simulink model "FlightModel"  (R2024b)
settings: Solver=ode1  StartTime=0.0  StopTime=inf  FixedStep=sampletime  RelTol=1e-3
values from neighbouring files (symbols this model uses):
  g = 9.807    [start.m]
undefined symbols (not defined in the file or in its folder): INI
settings Model: Creator=Nguewo  LastModifiedBy=annaf
settings SolverCC: AlgebraicLoopSolver=TrustRegion
settings DebuggingCC: UnconnectedInputMsg=warning  UnconnectedOutputMsg=warning  UnconnectedLineMsg=warning
settings ModelReferenceCC: EnableRefExpFcnMdlSchedulingChecks=on
settings RTWCC: GPUComputeCapability=3.5  DLArmComputeVersion=19.05

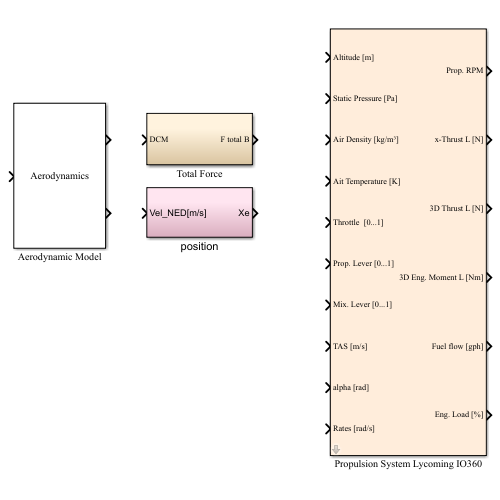
[thumbnail: Simulink's stored preview of the top-level diagram]
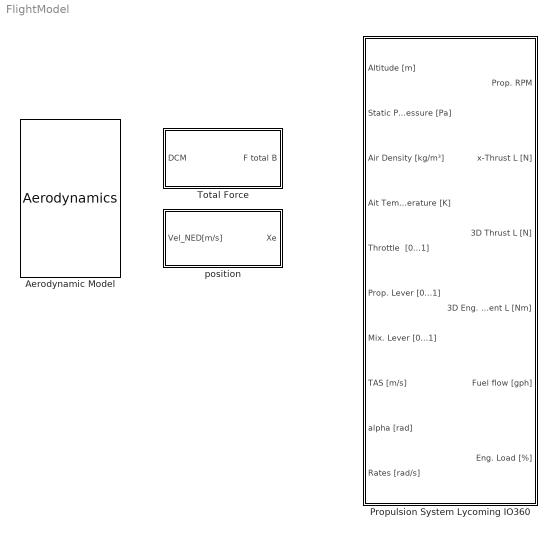
== system FlightModel ==
  Aerodynamic Model : M-S-Function  FunctionName=Aerodynamics
  Propulsion System Lycoming IO360 : Subsystem  mask{Y_TW=0}
      mask prompts: Y_TW "Y Position of the Engine [m]. Positive for Left Engine"
  Total Force : Subsystem
  position : Subsystem

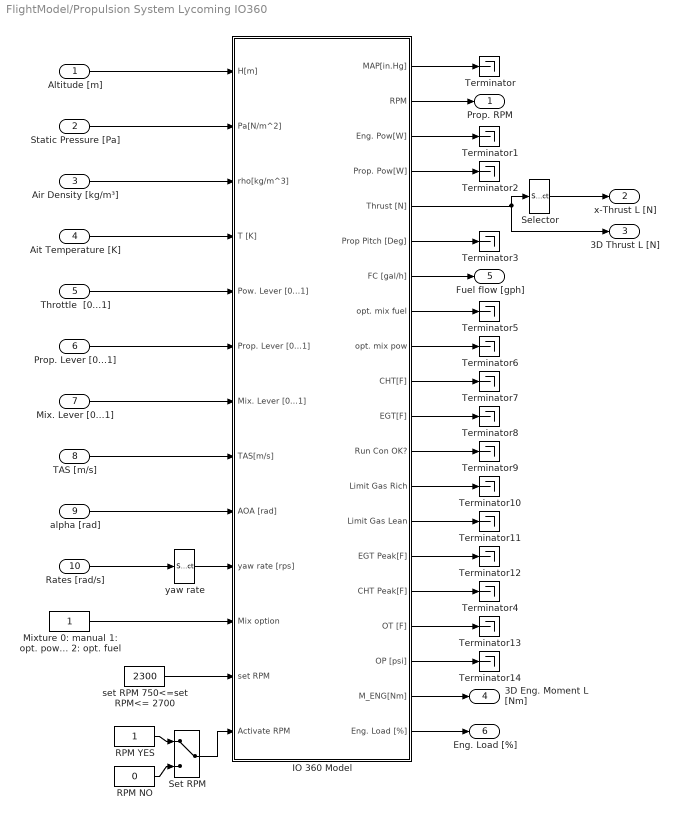
== system FlightModel/Propulsion System Lycoming IO360 ==
  Altitude [m] : Inport
  Static Pressure [Pa] : Inport  Port=2
  Air Density [kg/m³] : Inport  Port=3
  Ait Temperature [K] : Inport  Port=4
  Throttle  [0...1] : Inport  Port=5
  Prop. Lever [0...1] : Inport  Port=6
  Mix. Lever [0...1] : Inport  Port=7
  TAS [m/s] : Inport  Port=8
  alpha [rad] : Inport  Port=9
  Rates [rad/s] : Inport  Port=10
  IO 360 Model : Subsystem
  "Mixture 0: manual 1: opt. pow 2: opt. fuel " : Constant
  RPM NO : Constant  Value=0
  RPM YES : Constant
  Selector : Selector  InputPortWidth=3  IndexOptions=Index vector (dialog)  Indices=1  OutputSizes=1
  Set RPM : ManualSwitch
  Terminator{,1..14} (15 alike) : Terminator
  set RPM 750<=set RPM<= 2700 : Constant  Value=2300
  yaw rate : Selector  InputPortWidth=3  IndexOptions=Index vector (dialog)  Indices=3  OutputSizes=1
  Prop. RPM : Outport  VectorParamsAs1DForOutWhenUnconnected=off
  x-Thrust L [N] : Outport  Port=2  VectorParamsAs1DForOutWhenUnconnected=off
  3D Thrust L [N] : Outport  Port=3  VectorParamsAs1DForOutWhenUnconnected=off
  3D Eng. Moment L [Nm] : Outport  Port=4  VectorParamsAs1DForOutWhenUnconnected=off
  Fuel flow [gph] : Outport  Port=5  VectorParamsAs1DForOutWhenUnconnected=off
  Eng. Load [%] : Outport  Port=6  VectorParamsAs1DForOutWhenUnconnected=off
  wires:
  Selector/1 -> x-Thrust L [N]/1
  IO 360 Model/5(Thrust [N]) -> Selector/1, 3D Thrust L [N]/1
  IO 360 Model/19(M_ENG[Nm]) -> 3D Eng. Moment L [Nm]/1
  IO 360 Model/2(RPM) -> Prop. RPM/1
  IO 360 Model/1(MAP[in.Hg]) -> Terminator/1
  IO 360 Model/3(Eng. Pow[W]) -> Terminator1/1
  IO 360 Model/4(Prop. Pow[W]) -> Terminator2/1
  IO 360 Model/6(Prop Pitch [Deg]) -> Terminator3/1
  IO 360 Model/7(FC [gal/h]) -> Fuel flow [gph]/1
  IO 360 Model/8(opt. mix fuel) -> Terminator5/1
  IO 360 Model/9(opt. mix pow) -> Terminator6/1
  IO 360 Model/10(CHT[F]) -> Terminator7/1
  IO 360 Model/11(EGT[F]) -> Terminator8/1
  IO 360 Model/12(Run Con OK?) -> Terminator9/1
  IO 360 Model/13(Limit Gas Rich) -> Terminator10/1
  IO 360 Model/14(Limit Gas Lean) -> Terminator11/1
  IO 360 Model/15(EGT Peak[F]) -> Terminator12/1
  IO 360 Model/16(CHT Peak[F]) -> Terminator4/1
  IO 360 Model/17(OT [F]) -> Terminator13/1
  IO 360 Model/18(OP [psi]) -> Terminator14/1
  IO 360 Model/20(Eng. Load [%]) -> Eng. Load [%]/1
  Throttle  [0...1]/1 -> IO 360 Model/5(Pow. Lever [0...1])
  TAS [m/s]/1 -> IO 360 Model/8(TAS[m/s])
  Prop. Lever [0...1]/1 -> IO 360 Model/6(Prop. Lever [0...1])
  Mix. Lever [0...1]/1 -> IO 360 Model/7(Mix. Lever [0...1])
  alpha [rad]/1 -> IO 360 Model/9("AOA [rad] ")
  "Mixture 0: manual 1: opt. pow 2: opt. fuel "/1 -> IO 360 Model/11(Mix option)
  yaw rate/1 -> IO 360 Model/10(yaw rate [rps])
  Rates [rad/s]/1 -> yaw rate/1
  RPM NO/1 -> Set RPM/2
  RPM YES/1 -> Set RPM/1
  set RPM 750<=set RPM<= 2700/1 -> IO 360 Model/12(set RPM)
  Set RPM/1 -> IO 360 Model/13(Activate RPM)
  Altitude [m]/1 -> IO 360 Model/1(H[m])
  Static Pressure [Pa]/1 -> IO 360 Model/2(Pa[N/m^2])
  Air Density [kg/m³]/1 -> IO 360 Model/3(rho[kg/m^3])
  Ait Temperature [K]/1 -> IO 360 Model/4(T [K])

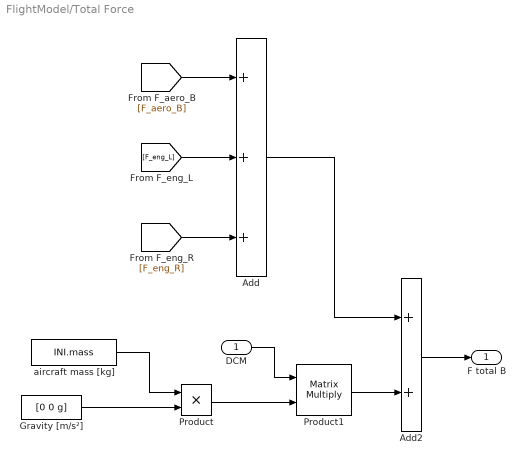
== system FlightModel/Total Force ==
  DCM : Inport
  Add : Sum  Inputs=+++
  Add2 : Sum
  Gravity [m/s²] : Constant  Value=[0 0 g]
  Product : Product
  Product1 : Product  Multiplication=Matrix(*)
  aircraft mass [kg] : Constant  Value=INI.mass
  F total B : Outport  VectorParamsAs1DForOutWhenUnconnected=off
  wires:
  Add/1 -> Add2/1
  Gravity [m/s²]/1 -> Product/2
  Product1/1 -> Add2/2
  Add2/1 -> F total B/1
  Product/1 -> Product1/2
  aircraft mass [kg]/1 -> Product/1
  DCM/1 -> Product1/1
  [F_eng_R] -> Add/3
  [F_eng_L] -> Add/2
  [F_aero_B] -> Add/1

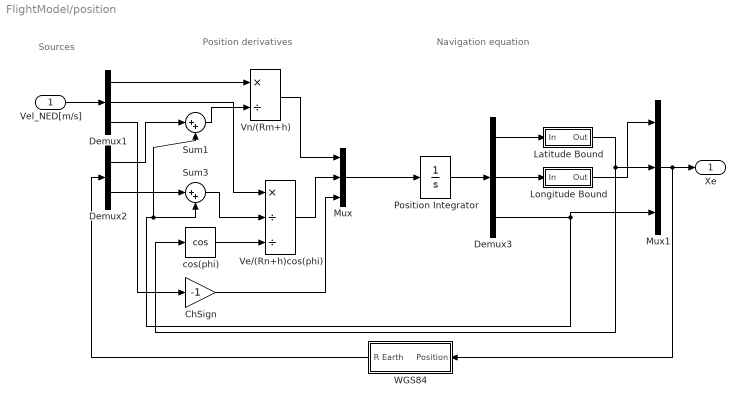
== system FlightModel/position ==
  note: Navigation equation
  note: Position derivatives
  note: Sources
  Vel_NED[m/s] : Inport
  ChSign : Gain  Gain=-1  SaturateOnIntegerOverflow=on  OutDataTypeStr=Inherit: Same as input  ParamDataTypeStr=Inherit: Same as input
  Demux1 : Demux  Outputs=3
      settings: DisplayOption=none
  Demux2 : Demux  Outputs=2
      settings: DisplayOption=none
  Demux3 : Demux  Outputs=3
      settings: DisplayOption=none
  Latitude Bound : Subsystem
  Longitude Bound : Subsystem
  Mux : Mux  Inputs=3
  Mux1 : Mux  Inputs=3
  Position Integrator : Integrator  InitialCondition=INI.POS
  Sum1 : Sum  Inputs=|++
  Sum3 : Sum  Inputs=|++
  Ve/(Rn+h)cos(phi) : Product  Inputs=*//  InputSameDT=on  SaturateOnIntegerOverflow=on  OutDataTypeStr=Inherit: Same as first input
  Vn/(Rm+h) : Product  Inputs=*/  InputSameDT=on  SaturateOnIntegerOverflow=on  OutDataTypeStr=Inherit: Same as first input
  WGS84 : Subsystem
  cos(phi) : Trigonometry  Operator=cos
  Xe : Outport  VectorParamsAs1DForOutWhenUnconnected=off
  wires:
  Longitude Bound/1(Out) -> Mux1/1
  Mux1/1 -> Xe/1, WGS84/1(Position)
  cos(phi)/1 -> Ve/(Rn+h)cos(phi)/3
  Demux3/1 -> Latitude Bound/1(In)
  ChSign/1 -> Mux/3
  Latitude Bound/1(Out) -> cos(phi)/1, Mux1/2
  Vn/(Rm+h)/1 -> Mux/1
  Demux1/2 -> Ve/(Rn+h)cos(phi)/1
  Demux1/1 -> Vn/(Rm+h)/1
  Vel_NED[m/s]/1 -> Demux1/1
  Demux1/3 -> ChSign/1
  Demux3/2 -> Longitude Bound/1(In)
  Demux3/3 -> Mux1/3, Sum3/2, Sum1/2
  Ve/(Rn+h)cos(phi)/1 -> Mux/2
  WGS84/1(R Earth) -> Demux2/1
  Sum1/1 -> Vn/(Rm+h)/2
  Demux2/1 -> Sum1/1
  Demux2/2 -> Sum3/1
  Sum3/1 -> Ve/(Rn+h)cos(phi)/2
  Position Integrator/1 -> Demux3/1
  Mux/1 -> Position Integrator/1

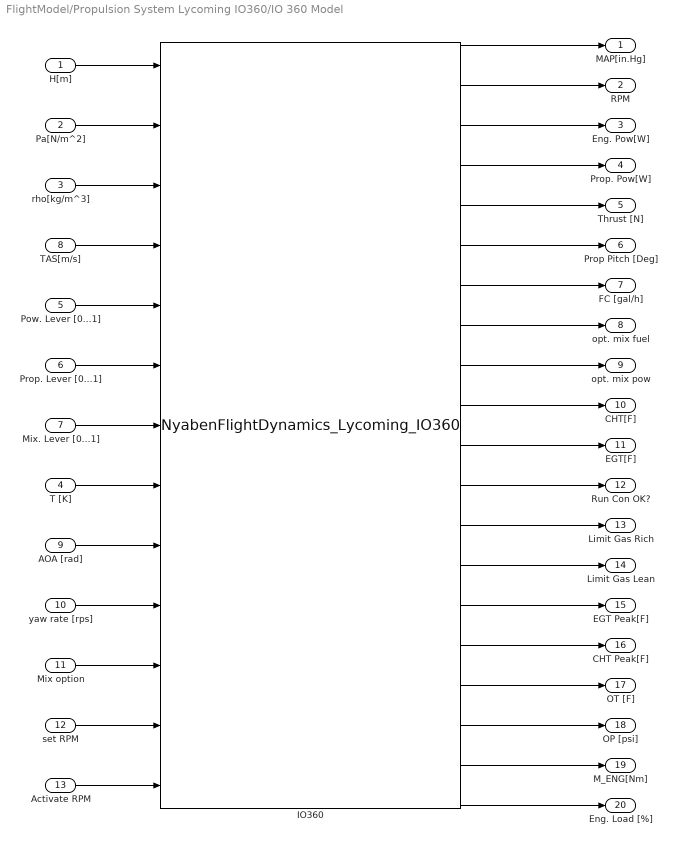
== system FlightModel/Propulsion System Lycoming IO360/IO 360 Model ==
  H[m] : Inport
  Pa[N/m^2] : Inport  Port=2
  rho[kg/m^3] : Inport  Port=3
  T [K] : Inport  Port=4
  Pow. Lever [0...1] : Inport  Port=5
  Prop. Lever [0...1] : Inport  Port=6
  Mix. Lever [0...1] : Inport  Port=7
  TAS[m/s] : Inport  Port=8
  "AOA [rad] " : Inport  Port=9
  yaw rate [rps] : Inport  Port=10
  Mix option : Inport  Port=11
  set RPM : Inport  Port=12
  Activate RPM : Inport  Port=13
  IO360 : S-Function  FunctionName=NyabenFlightDynamics_Lycoming_IO360  Parameters=Y_TW  SFunctionDeploymentMode=off  EnableBusSupport=off
  MAP[in.Hg] : Outport  VectorParamsAs1DForOutWhenUnconnected=off
  RPM : Outport  Port=2  VectorParamsAs1DForOutWhenUnconnected=off
  Eng. Pow[W] : Outport  Port=3  VectorParamsAs1DForOutWhenUnconnected=off
  Prop. Pow[W] : Outport  Port=4  VectorParamsAs1DForOutWhenUnconnected=off
  Thrust [N] : Outport  Port=5  VectorParamsAs1DForOutWhenUnconnected=off
  Prop Pitch [Deg] : Outport  Port=6  VectorParamsAs1DForOutWhenUnconnected=off
  FC [gal/h] : Outport  Port=7  VectorParamsAs1DForOutWhenUnconnected=off
  opt. mix fuel : Outport  Port=8  VectorParamsAs1DForOutWhenUnconnected=off
  opt. mix pow : Outport  Port=9  VectorParamsAs1DForOutWhenUnconnected=off
  CHT[F] : Outport  Port=10  VectorParamsAs1DForOutWhenUnconnected=off
  EGT[F] : Outport  Port=11  VectorParamsAs1DForOutWhenUnconnected=off
  Run Con OK? : Outport  Port=12  VectorParamsAs1DForOutWhenUnconnected=off
  Limit Gas Rich : Outport  Port=13  VectorParamsAs1DForOutWhenUnconnected=off
  Limit Gas Lean : Outport  Port=14  VectorParamsAs1DForOutWhenUnconnected=off
  EGT Peak[F] : Outport  Port=15  VectorParamsAs1DForOutWhenUnconnected=off
  CHT Peak[F] : Outport  Port=16  VectorParamsAs1DForOutWhenUnconnected=off
  OT [F] : Outport  Port=17  VectorParamsAs1DForOutWhenUnconnected=off
  OP [psi] : Outport  Port=18  VectorParamsAs1DForOutWhenUnconnected=off
  M_ENG[Nm] : Outport  Port=19  VectorParamsAs1DForOutWhenUnconnected=off
  Eng. Load [%] : Outport  Port=20  VectorParamsAs1DForOutWhenUnconnected=off
  wires:
  T [K]/1 -> IO360/8
  Mix. Lever [0...1]/1 -> IO360/7
  Prop. Lever [0...1]/1 -> IO360/6
  Pow. Lever [0...1]/1 -> IO360/5
  TAS[m/s]/1 -> IO360/4
  rho[kg/m^3]/1 -> IO360/3
  Pa[N/m^2]/1 -> IO360/2
  H[m]/1 -> IO360/1
  IO360/1 -> MAP[in.Hg]/1
  IO360/2 -> RPM/1
  IO360/3 -> Eng. Pow[W]/1
  IO360/4 -> Prop. Pow[W]/1
  IO360/5 -> Thrust [N]/1
  IO360/6 -> Prop Pitch [Deg]/1
  IO360/7 -> FC [gal/h]/1
  IO360/8 -> opt. mix fuel/1
  IO360/9 -> opt. mix pow/1
  IO360/10 -> CHT[F]/1
  IO360/11 -> EGT[F]/1
  IO360/12 -> Run Con OK?/1
  IO360/13 -> Limit Gas Rich/1
  IO360/14 -> Limit Gas Lean/1
  IO360/15 -> EGT Peak[F]/1
  IO360/16 -> CHT Peak[F]/1
  IO360/17 -> OT [F]/1
  IO360/18 -> OP [psi]/1
  IO360/19 -> M_ENG[Nm]/1
  yaw rate [rps]/1 -> IO360/10
  "AOA [rad] "/1 -> IO360/9
  Mix option/1 -> IO360/11
  set RPM/1 -> IO360/12
  Activate RPM/1 -> IO360/13
  IO360/20 -> Eng. Load [%]/1

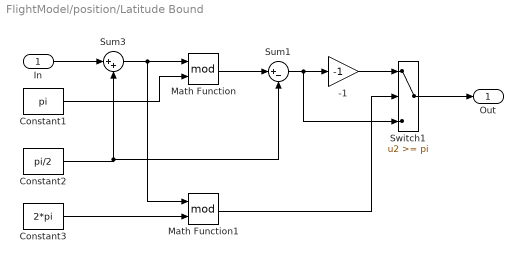
== system FlightModel/position/Latitude Bound ==
  In : Inport
  -1 : Gain  Gain=-1  SaturateOnIntegerOverflow=on  OutDataTypeStr=Inherit: Same as input  ParamDataTypeStr=Inherit: Same as input
  Constant1 : Constant  Value=pi
  Constant2 : Constant  Value=pi/2
  Constant3 : Constant  Value=2*pi
  Math Function : Math  Operator=mod  SignedPower=on
  Math Function1 : Math  Operator=mod  SignedPower=on
  Sum1 : Sum  Inputs=|+-
  Sum3 : Sum  Inputs=|++
  Switch1 : Switch  Threshold=pi  SaturateOnIntegerOverflow=off  InputSameDT=off
  Out : Outport  VectorParamsAs1DForOutWhenUnconnected=off
  wires:
  -1/1 -> Switch1/1
  Switch1/1 -> Out/1
  Math Function/1 -> Sum1/1
  Sum1/1 -> Switch1/3, -1/1
  Constant3/1 -> Math Function1/2
  Constant2/1 -> Sum1/2, Sum3/2
  Constant1/1 -> Math Function/2
  In/1 -> Sum3/1
  Math Function1/1 -> Switch1/2
  Sum3/1 -> Math Function1/1, Math Function/1

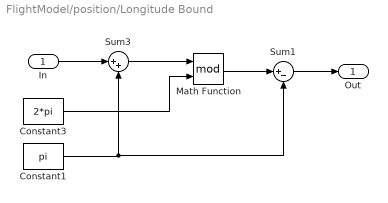
== system FlightModel/position/Longitude Bound ==
  In : Inport
  Constant1 : Constant  Value=pi
  Constant3 : Constant  Value=2*pi
  Math Function : Math  Operator=mod  SignedPower=on
  Sum1 : Sum  Inputs=|+-
  Sum3 : Sum  Inputs=|++
  Out : Outport  VectorParamsAs1DForOutWhenUnconnected=off
  wires:
  Sum3/1 -> Math Function/1
  In/1 -> Sum3/1
  Constant1/1 -> Sum1/2, Sum3/2
  Constant3/1 -> Math Function/2
  Math Function/1 -> Sum1/1
  Sum1/1 -> Out/1

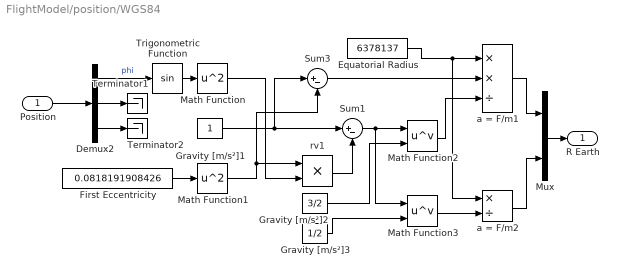
== system FlightModel/position/WGS84 ==
  Position : Inport
  Demux2 : Demux  Outputs=3
  Equatorial Radius : Constant  Value=6378137
  First Eccentricity : Constant  Value=0.0818191908426
  Gravity [m/s²]1 : Constant
  Gravity [m/s²]2 : Constant  Value=3/2
  Gravity [m/s²]3 : Constant  Value=1/2
  Math Function : Math  Operator=square  SignedPower=on
  Math Function1 : Math  Operator=square  SignedPower=on
  Math Function2 : Math  Operator=pow  SignedPower=on
  Math Function3 : Math  Operator=pow  SignedPower=on
  Mux : Mux  Inputs=2
  Sum1 : Sum  Inputs=|+-
  Sum3 : Sum  Inputs=|+-
  Terminator1 : Terminator
  Terminator2 : Terminator
  Trigonometric Function : Trigonometry
  a = F/m1 : Product  Inputs=**/
  a = F/m2 : Product  Inputs=*/
  rv1 : Product
  R Earth : Outport  VectorParamsAs1DForOutWhenUnconnected=off
  wires:
  Gravity [m/s²]2/1 -> Math Function2/2
  a = F/m2/1 -> Mux/2
  Gravity [m/s²]3/1 -> Math Function3/2
  Math Function3/1 -> a = F/m2/2
  First Eccentricity/1 -> Math Function1/1
  Math Function1/1 -> Sum3/2, rv1/1
  Trigonometric Function/1 -> Math Function/1
  rv1/1 -> Sum1/2
  Sum1/1 -> Math Function3/1, Math Function2/1
  Position/1 -> Demux2/1
  Demux2/1 -> Trigonometric Function/1  "phi"
  Demux2/3 -> Terminator2/1
  Demux2/2 -> Terminator1/1
  a = F/m1/1 -> Mux/1
  Math Function/1 -> rv1/2
  Math Function2/1 -> a = F/m1/3
  Equatorial Radius/1 -> a = F/m2/1, a = F/m1/1
  Sum3/1 -> a = F/m1/2
  Gravity [m/s²]1/1 -> Sum1/1, Sum3/1
  Mux/1 -> R Earth/1
